simulink model "test_state_space"  (R2022b)
settings: Solver=ode5  StartTime=0.0  StopTime=30  FixedStep=0.01  RelTol=1e-3
settings Model: Creator=jonas  LastModifiedBy=jonas
settings DebuggingCC: UnderSpecifiedDimensionMsg=warning

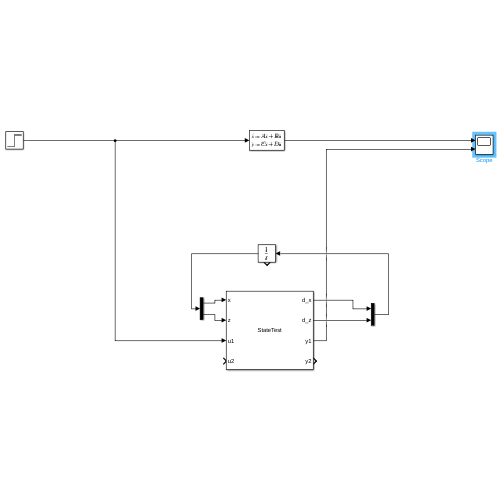
[thumbnail: Simulink's stored preview of the top-level diagram]
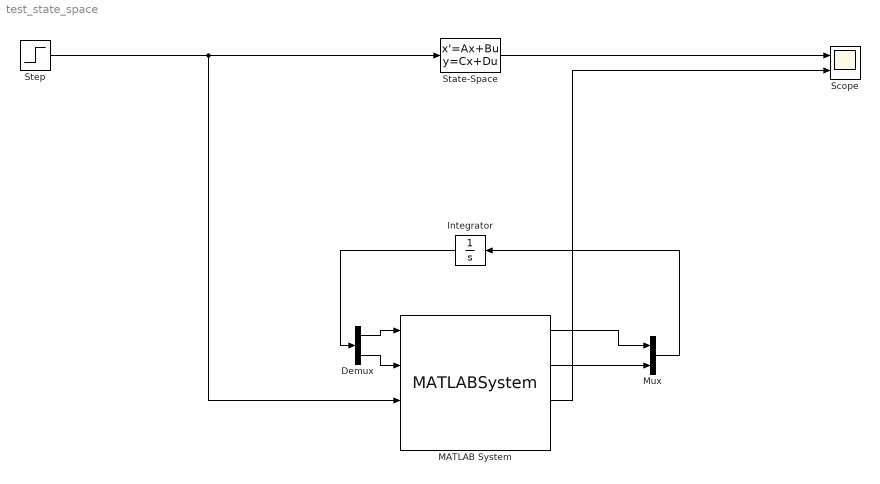
== system test_state_space ==
  Demux : Demux  Outputs=2
  Integrator : Integrator  ShowStatePort=on
  MATLAB System : MATLABSystem  System=StateTest  m=1.0  C=-1  SimulateUsing=Code generation
      mask Type: StateTest
      mask Display:
      | disp('StateTest');
      | port_label('input',1,'x');
      | port_label('input',2,'z');
      | port_label('input',3,'u1');
      | port_label('input',4,'u2');
      | port_label('output',1,'d_x');
      | port_label('output',2,'d_z');
      | port_label('output',3,'y1');
      | port_label('output',4,'y2');
  Mux : Mux  Inputs=2
  Scope : Scope  NumInputPorts=2
  State-Space : StateSpace  A=[0 1 ; -1 -1]  B=[0 ; 1]  C=[1 0]  D=0  InitialCondition=0  ParameterTunability=Unconstrained
  Step : Step  SampleTime=0
  wires:
  Step/1 -> MATLAB System/3, State-Space/1
  State-Space/1 -> Scope/1
  MATLAB System/3 -> Scope/2
  MATLAB System/1 -> Mux/1
  MATLAB System/2 -> Mux/2
  Mux/1 -> Integrator/1
  Demux/1 -> MATLAB System/1
  Demux/2 -> MATLAB System/2
  Integrator/1 -> Demux/1
